simulink model "input_tf"  (Simulink 7.4)
settings: Solver=ode45  StartTime=0.0  StopTime=10.0  RelTol=1e-3
values from neighbouring files (symbols this model uses):
  Gd = 1    [a2_data_input_examsim1.m]
undefined symbols (not defined in the file or in its folder): dp_coeff, dp_freq, dp_type
settings Model: Creator=Vittorio  LastModifiedBy=Vittorio

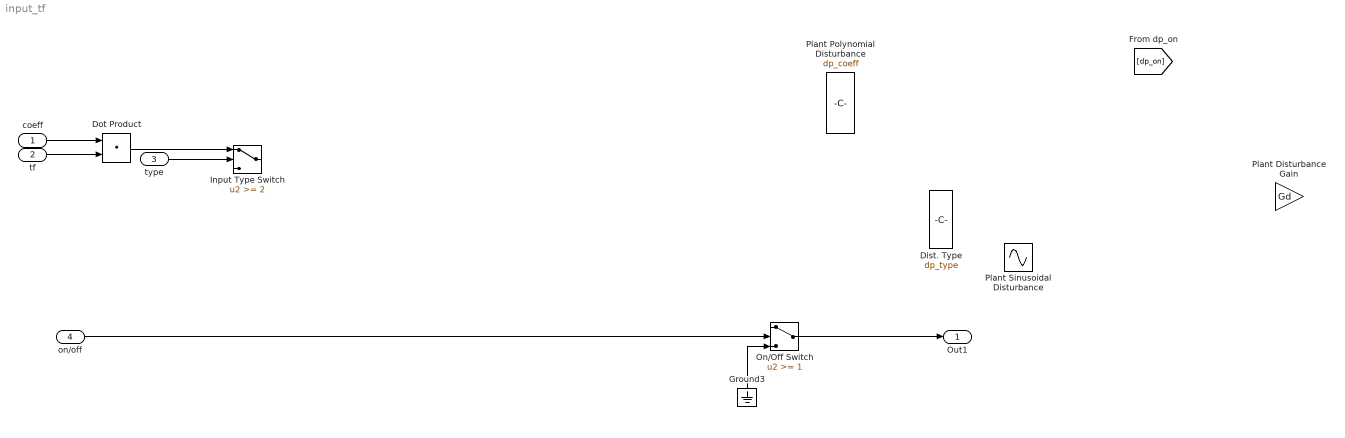
== system input_tf ==
  coeff : Inport  OutDataType=fixdt(1, 16)  OutScaling=2^0
  tf : Inport  Port=2  OutDataType=fixdt(1, 16)  OutScaling=2^0
  type : Inport  Port=3  OutDataType=fixdt(1, 16)  OutScaling=2^0
  on/off : Inport  Port=4  OutDataType=fixdt(1, 16)  OutScaling=2^0
  Dist. Type : Constant  Value=dp_type
  Dot Product : DotProduct  OutDataType=fixdt(1, 16)  OutScaling=2^-10  InputSameDT=on  OutDataTypeStr=Inherit: Inherit via internal rule
  Ground3 : Ground
  Input Type Switch : Switch  Threshold=2
  On/Off Switch : Switch  Threshold=1
  Plant Disturbance Gain : Gain  Gain=Gd
  Plant Polynomial Disturbance : Constant  Value=dp_coeff
  Plant Sinusoidal Disturbance : Sin  Amplitude=dp_coeff  Bias=0  Frequency=dp_freq  Phase=0  Samples=10  SampleTime=0  Offset=0
  Out1 : Outport  OutDataType=fixdt(1, 16)  OutScaling=2^0
  wires:
  Ground3/1 -> On/Off Switch/3
  on/off/1 -> On/Off Switch/2
  On/Off Switch/1 -> Out1/1
  coeff/1 -> Dot Product/1
  tf/1 -> Dot Product/2
  Dot Product/1 -> Input Type Switch/1
  type/1 -> Input Type Switch/2
